simulink library "UDP_Communication"  (R2016b)
settings: Solver=VariableStepAuto  StartTime=0.0  StopTime=10.0  RelTol=1e-3
undefined symbols (not defined in the file): CassieParameters
libraries: UDP_Communication x12, xpcutilitieslib x6, xpcrtudplib x6, StateEstimation x2
settings Model: Creator=Ross Hartley  LastModifiedBy=Ross Hartley

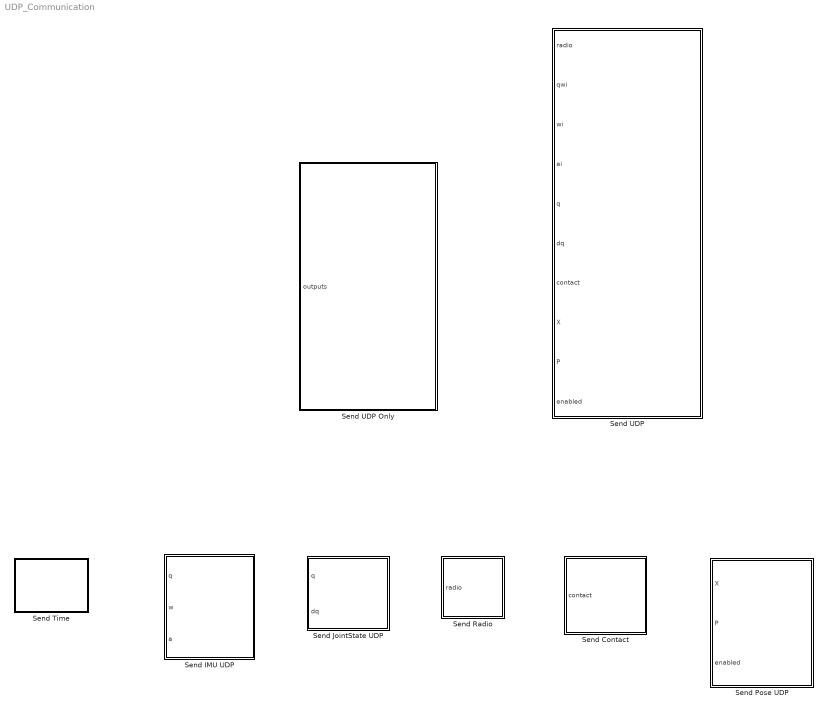
== system UDP_Communication ==
  Send Contact : Subsystem
  Send IMU UDP : Subsystem
  Send JointState UDP : Subsystem
  Send Pose UDP : Subsystem
  Send Radio : Subsystem
  Send Time : Subsystem
  Send UDP : Subsystem
  Send UDP Only : Subsystem

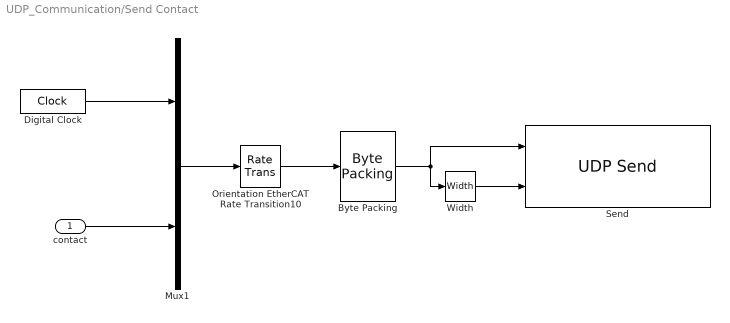
== system UDP_Communication/Send Contact ==
  contact : Inport
  "Byte Packing " : xpcutilitieslib/Byte Packing   MaskPackedDataType=uint8  MaskUnpackedDataTypes={'double'}  MaskAlignment=1
  Digital Clock : DigitalClock  SampleTime=CassieParameters.etherCatSampleTime
  Mux1 : Mux  Inputs=2
  Orientation EtherCAT Rate Transition10 : RateTransition  Deterministic=off  OutPortSampleTime=Contact_UDP_SampleTime
  Send : xpcrtudplib/UDP Send  ipAddressVal=Use host-target connection  localPort=-1  toAddress=10.10.10.5  toPort=25004  sampleTime=Contact_UDP_SampleTime
  Width : Width
  wires:
  contact/1 -> Mux1/2
  Digital Clock/1 -> Mux1/1
  Orientation EtherCAT Rate Transition10/1 -> "Byte Packing "/1
  Width/1 -> Send/2
  "Byte Packing "/1 -> Send/1, Width/1
  Mux1/1 -> Orientation EtherCAT Rate Transition10/1

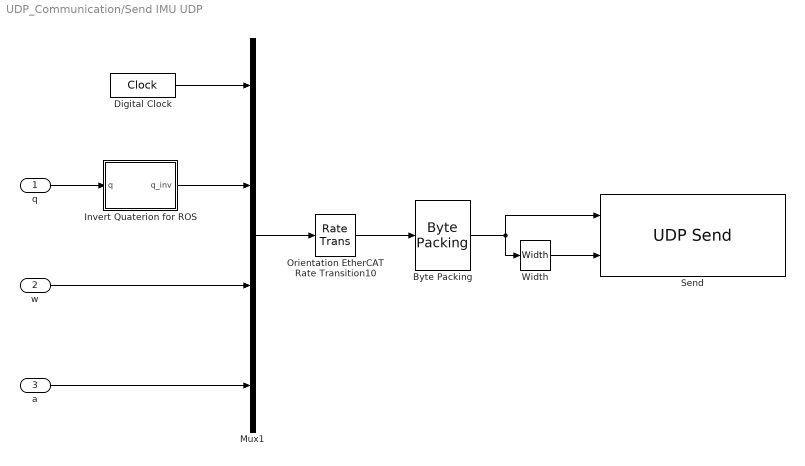
== system UDP_Communication/Send IMU UDP ==
  q : Inport
  w : Inport  Port=2
  a : Inport  Port=3
  "Byte Packing " : xpcutilitieslib/Byte Packing   MaskPackedDataType=uint8  MaskUnpackedDataTypes={'double'}  MaskAlignment=1
  Digital Clock : DigitalClock  SampleTime=CassieParameters.etherCatSampleTime
  Invert Quaterion for ROS : MATLAB Function  TreatAsAtomicUnit=on
  Mux1 : Mux
  Orientation EtherCAT Rate Transition10 : RateTransition  Deterministic=off  OutPortSampleTime=IMU_UDP_SampleTime
  Send : xpcrtudplib/UDP Send  ipAddressVal=Use host-target connection  localPort=-1  toAddress=10.10.10.5  toPort=25001  sampleTime=IMU_UDP_SampleTime
  Width : Width
  wires:
  Mux1/1 -> Orientation EtherCAT Rate Transition10/1
  "Byte Packing "/1 -> Width/1, Send/1
  Width/1 -> Send/2
  Orientation EtherCAT Rate Transition10/1 -> "Byte Packing "/1
  Digital Clock/1 -> Mux1/1
  a/1 -> Mux1/4
  q/1 -> Invert Quaterion for ROS/1(q)
  w/1 -> Mux1/3
  Invert Quaterion for ROS/1(q_inv) -> Mux1/2

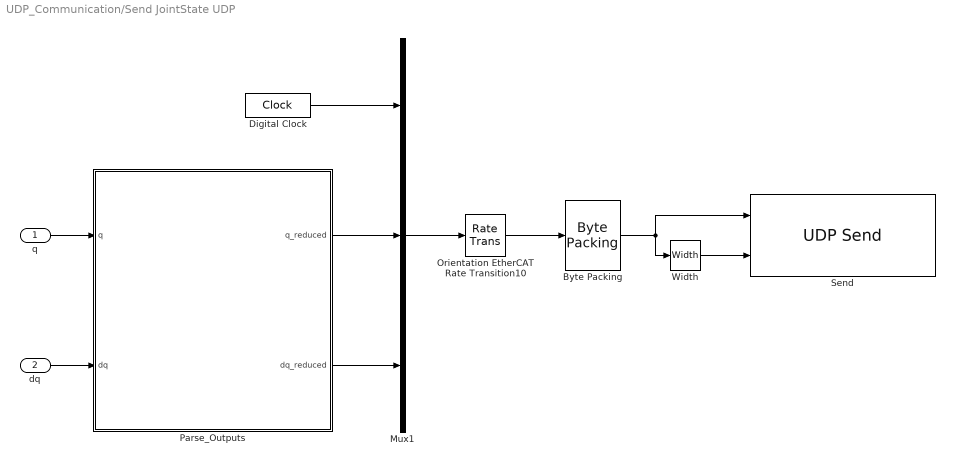
== system UDP_Communication/Send JointState UDP ==
  q : Inport
  dq : Inport  Port=2
  "Byte Packing " : xpcutilitieslib/Byte Packing   MaskPackedDataType=uint8  MaskUnpackedDataTypes={'double'}  MaskAlignment=1
  Digital Clock : DigitalClock  SampleTime=CassieParameters.etherCatSampleTime
  Mux1 : Mux  Inputs=3
  Orientation EtherCAT Rate Transition10 : RateTransition  Deterministic=off  OutPortSampleTime=JointState_UDP_SampleTime
  Parse_Outputs : MATLAB Function  TreatAsAtomicUnit=on
  Send : xpcrtudplib/UDP Send  ipAddressVal=Use host-target connection  localPort=-1  toAddress=10.10.10.5  toPort=25002  sampleTime=JointState_UDP_SampleTime
  Width : Width
  wires:
  Mux1/1 -> Orientation EtherCAT Rate Transition10/1
  "Byte Packing "/1 -> Width/1, Send/1
  Width/1 -> Send/2
  Orientation EtherCAT Rate Transition10/1 -> "Byte Packing "/1
  Digital Clock/1 -> Mux1/1
  Parse_Outputs/1(q_reduced) -> Mux1/2
  Parse_Outputs/2(dq_reduced) -> Mux1/3
  dq/1 -> Parse_Outputs/2(dq)
  q/1 -> Parse_Outputs/1(q)

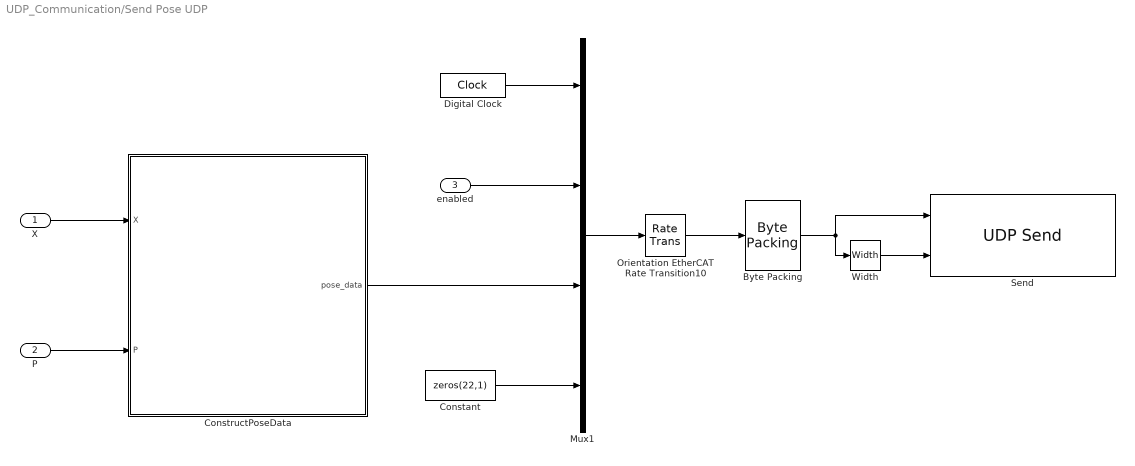
== system UDP_Communication/Send Pose UDP ==
  X : Inport
  P : Inport  Port=2
  enabled : Inport  Port=3
  "Byte Packing " : xpcutilitieslib/Byte Packing   MaskPackedDataType=uint8  MaskUnpackedDataTypes={'double'}  MaskAlignment=1
  Constant : Constant  Value=zeros(22,1)
  ConstructPoseData : MATLAB Function  TreatAsAtomicUnit=on
  Digital Clock : DigitalClock  SampleTime=CassieParameters.etherCatSampleTime
  Mux1 : Mux
  Orientation EtherCAT Rate Transition10 : RateTransition  Deterministic=off  OutPortSampleTime=Pose_UDP_SampleTime
  Send : xpcrtudplib/UDP Send  ipAddressVal=Use host-target connection  localPort=-1  toAddress=10.10.10.5  toPort=25000  sampleTime=Pose_UDP_SampleTime
  Width : Width
  wires:
  ConstructPoseData/1(pose_data) -> Mux1/3
  Digital Clock/1 -> Mux1/1
  enabled/1 -> Mux1/2
  P/1 -> ConstructPoseData/2(P)
  X/1 -> ConstructPoseData/1(X)
  Orientation EtherCAT Rate Transition10/1 -> "Byte Packing "/1
  Width/1 -> Send/2
  "Byte Packing "/1 -> Send/1, Width/1
  Mux1/1 -> Orientation EtherCAT Rate Transition10/1
  Constant/1 -> Mux1/4

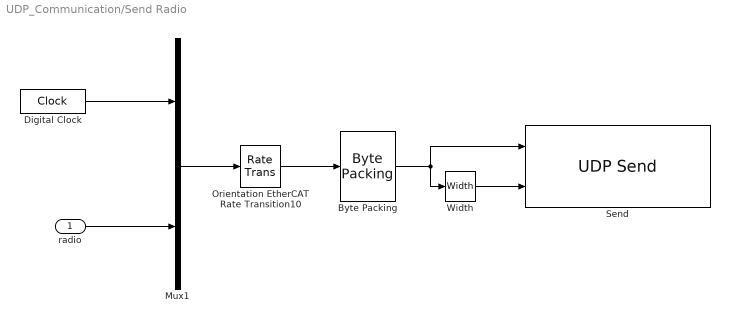
== system UDP_Communication/Send Radio ==
  radio : Inport
  "Byte Packing " : xpcutilitieslib/Byte Packing   MaskPackedDataType=uint8  MaskUnpackedDataTypes={'double'}  MaskAlignment=1
  Digital Clock : DigitalClock  SampleTime=CassieParameters.etherCatSampleTime
  Mux1 : Mux  Inputs=2
  Orientation EtherCAT Rate Transition10 : RateTransition  Deterministic=off  OutPortSampleTime=Radio_UDP_SampleTime
  Send : xpcrtudplib/UDP Send  ipAddressVal=Use host-target connection  localPort=-1  toAddress=10.10.10.5  toPort=25003  sampleTime=Radio_UDP_SampleTime
  Width : Width
  wires:
  Mux1/1 -> Orientation EtherCAT Rate Transition10/1
  "Byte Packing "/1 -> Width/1, Send/1
  Width/1 -> Send/2
  Orientation EtherCAT Rate Transition10/1 -> "Byte Packing "/1
  Digital Clock/1 -> Mux1/1
  radio/1 -> Mux1/2

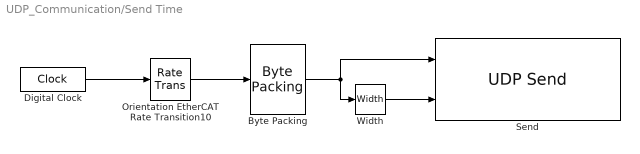
== system UDP_Communication/Send Time ==
  "Byte Packing " : xpcutilitieslib/Byte Packing   MaskPackedDataType=uint8  MaskUnpackedDataTypes={'double'}  MaskAlignment=1
  Digital Clock : DigitalClock  SampleTime=CassieParameters.etherCatSampleTime
  Orientation EtherCAT Rate Transition10 : RateTransition  Deterministic=off  OutPortSampleTime=Time_UDP_SampleTime
  Send : xpcrtudplib/UDP Send  ipAddressVal=Use host-target connection  localPort=-1  toAddress=10.10.10.105  toPort=25005  sampleTime=Time_UDP_SampleTime
  Width : Width
  wires:
  Digital Clock/1 -> Orientation EtherCAT Rate Transition10/1
  "Byte Packing "/1 -> Width/1, Send/1
  Width/1 -> Send/2
  Orientation EtherCAT Rate Transition10/1 -> "Byte Packing "/1

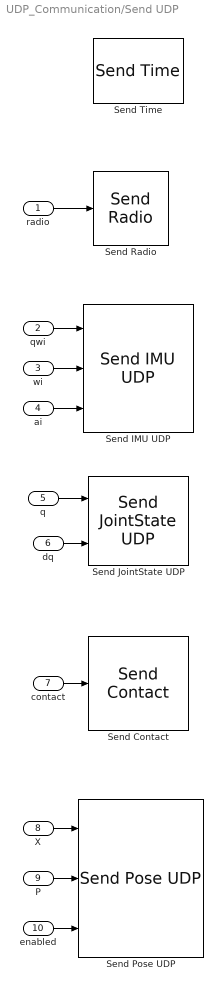
== system UDP_Communication/Send UDP ==
  radio : Inport
  qwi : Inport  Port=2
  wi : Inport  Port=3
  ai : Inport  Port=4
  q : Inport  Port=5
  dq : Inport  Port=6
  contact : Inport  Port=7
  X : Inport  Port=8
  P : Inport  Port=9
  enabled : Inport  Port=10
  Send Contact : UDP_Communication/Send Contact
  Send IMU UDP : UDP_Communication/Send IMU UDP
  Send JointState UDP : UDP_Communication/Send JointState UDP
  Send Pose UDP : UDP_Communication/Send Pose UDP
  Send Radio : UDP_Communication/Send Radio
  Send Time : UDP_Communication/Send Time
  wires:
  radio/1 -> Send Radio/1
  qwi/1 -> Send IMU UDP/1
  wi/1 -> Send IMU UDP/2
  ai/1 -> Send IMU UDP/3
  q/1 -> Send JointState UDP/1
  dq/1 -> Send JointState UDP/2
  contact/1 -> Send Contact/1
  X/1 -> Send Pose UDP/1
  P/1 -> Send Pose UDP/2
  enabled/1 -> Send Pose UDP/3

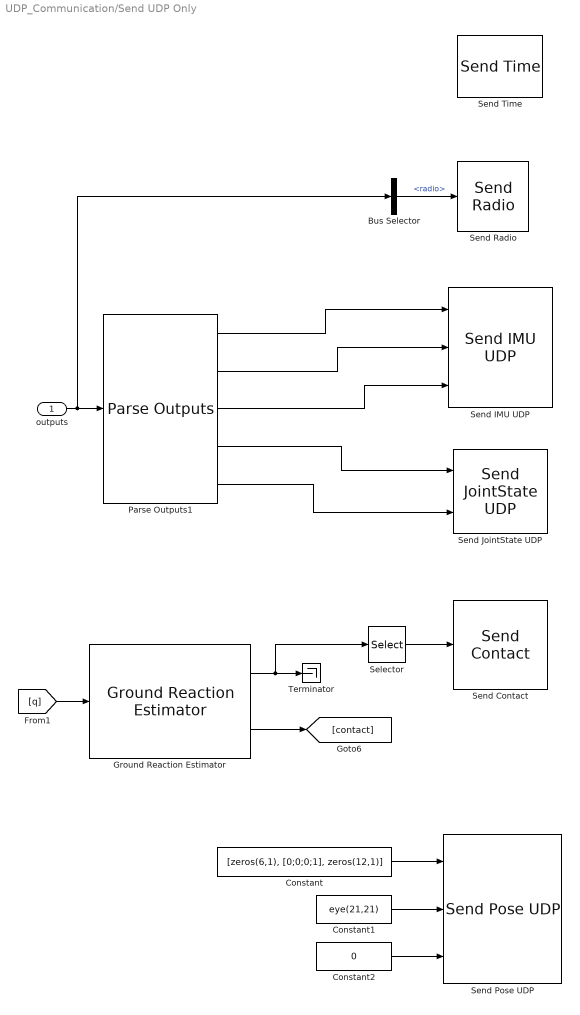
== system UDP_Communication/Send UDP Only ==
  outputs : Inport
  Bus Selector : BusSelector  OutputSignals=radio
  Constant : Constant  Value=[zeros(6,1), [0;0;0;1], zeros(12,1)]
  Constant1 : Constant  Value=eye(21,21)
  Constant2 : Constant  Value=0
  Ground Reaction Estimator : StateEstimation/Ground Reaction Estimator
  Parse Outputs1 : StateEstimation/Parse Outputs
  Selector : Selector  InputPortWidth=4  IndexOptions=Index vector (dialog)  Indices=[2, 4]  OutputSizes=1
  Send Contact : UDP_Communication/Send Contact
  Send IMU UDP : UDP_Communication/Send IMU UDP
  Send JointState UDP : UDP_Communication/Send JointState UDP
  Send Pose UDP : UDP_Communication/Send Pose UDP
  Send Radio : UDP_Communication/Send Radio
  Send Time : UDP_Communication/Send Time
  Terminator : Terminator
  wires:
  Constant/1 -> Send Pose UDP/1
  Constant1/1 -> Send Pose UDP/2
  Constant2/1 -> Send Pose UDP/3
  Ground Reaction Estimator/1 -> Selector/1, Terminator/1
  [q] -> Ground Reaction Estimator/1
  Ground Reaction Estimator/2 -> [contact]
  outputs/1 -> Bus Selector/1, Parse Outputs1/1
  Parse Outputs1/1 -> Send IMU UDP/1
  Parse Outputs1/3 -> Send IMU UDP/3
  Parse Outputs1/4 -> Send JointState UDP/1
  Parse Outputs1/5 -> Send JointState UDP/2
  Parse Outputs1/2 -> Send IMU UDP/2
  Bus Selector/1 -> Send Radio/1  "<radio>"
  Selector/1 -> Send Contact/1

== matlab function UDP_Communication/Send IMU UDP/Invert Quaterion for ROS ==
  data: q input; q_inv output
function q_inv = fcn(q)
    q_inv = Angles.Rotation_to_Quaternion( Angles.Quaternion_to_Rotation(q)' );
end

== matlab function UDP_Communication/Send JointState UDP/Parse_Outputs ==
  data: q_reduced output; dq_reduced output; q input; dq input
function [q_reduced, dq_reduced] = ReduceState(q, dq)
% Reduce state vector for use in ROS network

q_reduced = q(7:end);
dq_reduced = dq(7:end);

end

== matlab function UDP_Communication/Send Pose UDP/ConstructPoseData ==
  data: pose_data output; X input; P input
function pose_data = ConstructPoseData(X, P)
% Construct pose data for use in ROS network
% Publish everything in pelvis frame

% Rwi = X(1:3,1:3); 
% pose_data = zeros(43,1); 
% pose_data(1:3) = X(1:3,5) + Rwi*p_VectorNav_to_Pelvis(zeros(14,1));
% pose_data(4:7) = Angles.Rotation_to_Quaternion( (Rwi * R_VectorNav_to_Pelvis(zeros(14,1)))' );


Rwi = Angles.Quaternion_to_Rotation(X(7:10))';
pose_data = zeros(43,1); 
pose_data(1:3) = X(1:3) + Rwi*p_VectorNav_to_Pelvis(zeros(14,1));
pose_data(4:7) = Angles.Rotation_to_Quaternion( (Rwi * R_VectorNav_to_Pelvis(zeros(14,1)))' );


% TODO: Convert covariance of IMU pose to Body pose (Ross) 
pose_data(8:end) = reshape(P([1:3,1:3],[7:9,7:9]),[],1);

end
